simulink model "thinning1_131121"  (R2018b)
settings: Solver=FixedStepDiscrete  StartTime=0.0  StopTime=10.0  RelTol=1e-3
undefined symbols (not defined in the file or in its folder): gray
libraries: hdlsllib x2, visionsources x1, dspmtrx3 x1
settings Model: Creator=Administrator  LastModifiedBy=Administrator
settings OptimizationCC: BlockReduction=off  ConditionallyExecuteInputs=off  DefaultParameterBehavior=Inlined
settings DebuggingCC: AlgebraicLoopMsg=error  SingleTaskRateTransMsg=error
settings HardwareCC: ProdBitPerPointer=32  ProdBitPerSizeT=32  ProdBitPerPtrDiffT=32  ProdLargestAtomicFloat=None  ProdIntDivRoundTo=Undefined  ProdEndianess=Unspecified  ProdWordSize=32  ProdHWDeviceType=ASIC/FPGA->ASIC/FPGA  TargetBitPerPointer=64  TargetBitPerSizeT=64  TargetBitPerPtrDiffT=64  TargetLongLongMode=on  TargetIntDivRoundTo=Zero  TargetEndianess=LittleEndian  TargetWordSize=64  TargetHWDeviceType=Custom Processor->MATLAB Host Computer  ProdEqTarget=off

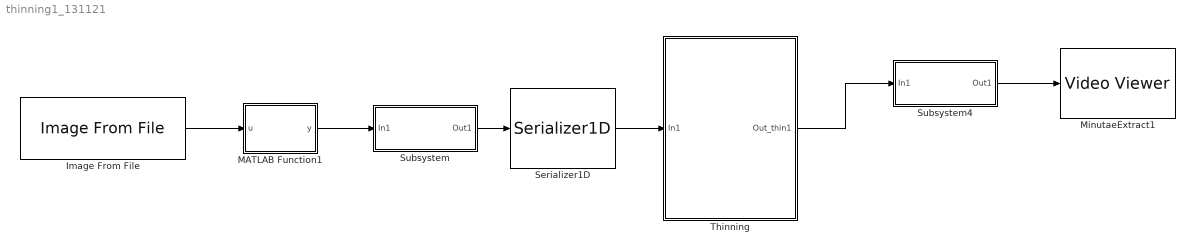
== system thinning1_131121 ==
  Image From File : visionsources/Image From File  Tag=vipblks_nd  FileName=C:\Users\Administrator\Desktop\chapter\101_4.tif  imagePorts=One multidimensional signal  Ts=0.1  ImageDataType=uint8  Signed=on  WordLength=16  sdImageDataType=uint(8)  FractionLengthMode=User-defined  FractionLength=15  OutPortLabels=R|G|B
      settings: SourceProductName=Computer Vision System Toolbox
  MATLAB Function1 : MATLAB Function  TreatAsAtomicUnit=on
  MinutaeExtract1 : VideoViewer  colormapValue=gray(256)  FigPos=[399 902 376 593]
  Serializer1D : hdlsllib/HDL Operations/Serializer1D  Ratio=1  IdleCycles=0  validIn=off  startOut=off  validOut=off  inputDataDimensions=8192  inputSampleTime=-1  inputSignalType=auto
      settings: SourceProductName=HDL Coder  SourceProductBaseCode=HD
  Subsystem : Subsystem
  Subsystem4 : Subsystem
  Thinning : Subsystem  TreatAsAtomicUnit=on
  wires:
  MATLAB Function1/1(y) -> Subsystem/1(In1)
  Image From File/1 -> MATLAB Function1/1(u)
  Subsystem/1(Out1) -> Serializer1D/1
  Serializer1D/1 -> Thinning/1(In1)
  Thinning/1(Out_thin1) -> Subsystem4/1(In1)
  Subsystem4/1(Out1) -> MinutaeExtract1/1

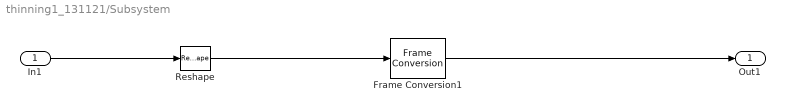
== system thinning1_131121/Subsystem ==
  In1 : Inport
  Frame Conversion1 : FrameConversion  OutFrame=Sample-based
  Reshape : Reshape
  Out1 : Outport
  wires:
  Frame Conversion1/1 -> Out1/1
  Reshape/1 -> Frame Conversion1/1
  In1/1 -> Reshape/1

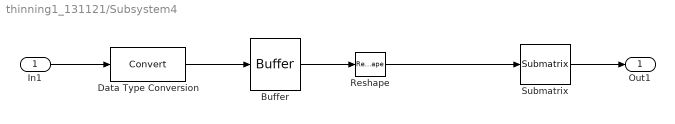
== system thinning1_131121/Subsystem4 ==
  In1 : Inport
  Buffer : Buffer  N=8192  OutputFrames=off
  Data Type Conversion : DataTypeConversion
  Reshape : Reshape  OutputDimensionality=Customize  OutputDimensions=[128,64]
  Submatrix : dspmtrx3/Submatrix  RowSpan=Range of rows  RowStartMode=First  RowStartIndex=1  RowEndMode=Last  RowEndIndex=1  ColSpan=Range of columns  ColStartMode=First  ColStartIndex=1  ColEndMode=Last  ColEndIndex=1
  Out1 : Outport
  wires:
  Data Type Conversion/1 -> Buffer/1
  Buffer/1 -> Reshape/1
  Reshape/1 -> Submatrix/1
  Submatrix/1 -> Out1/1
  In1/1 -> Data Type Conversion/1

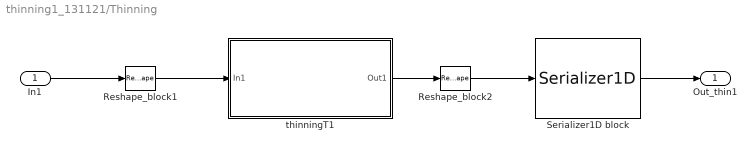
== system thinning1_131121/Thinning ==
  In1 : Inport
  Reshape_block1 : Reshape  OutputDimensionality=Customize  OutputDimensions=[128,64]
  Reshape_block2 : Reshape  OutputDimensionality=Column vector (2-D)  OutputDimensions=[128,64]
  Serializer1D block : hdlsllib/HDL Operations/Serializer1D  Ratio=8192  IdleCycles=0  validIn=off  startOut=off  validOut=off  inputDataDimensions=-1  inputSampleTime=-1  inputSignalType=auto
      settings: SourceProductName=HDL Coder  SourceProductBaseCode=HD
  thinningT1 : Subsystem  TreatAsAtomicUnit=on
  Out_thin1 : Outport
  wires:
  Reshape_block1/1 -> thinningT1/1(In1)
  In1/1 -> Reshape_block1/1
  Reshape_block2/1 -> Serializer1D block/1
  Serializer1D block/1 -> Out_thin1/1
  thinningT1/1(Out1) -> Reshape_block2/1

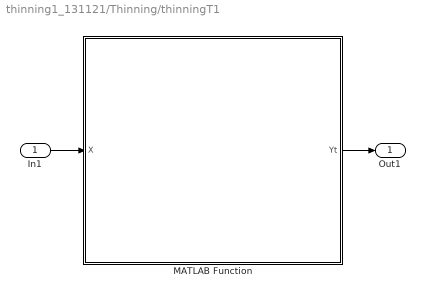
== system thinning1_131121/Thinning/thinningT1 ==
  In1 : Inport
  MATLAB Function : MATLAB Function  TreatAsAtomicUnit=on
  Out1 : Outport
  wires:
  In1/1 -> MATLAB Function/1(X)
  MATLAB Function/1(Yt) -> Out1/1

== matlab function thinning1_131121/MATLAB Function1 ==
  data: u input; y output
function y = fcn(u)
%#codegen
%i = rgb2gray(u);
b = u(100:227,150:213);
y = imbinarize(b);
%y = y(100:227,150:213);
%y = imbinarize(r);

== matlab function thinning1_131121/Thinning/thinningT1/MATLAB Function ==
  data: X input; Yt output
function Yt=thinningTh(X)
%img = imread ('2_4.jpg'); 
%Xr = rgb2gray(img);
%%%X = imbinarize(Xr);
%X = X(1:128,1:64);
[M,N]=size(X);
Yt = false(M,N);
Y=false(M,N,20);
Z=false(M,N,20);
Y(:,:,1)=X;
Z(:,:,1)=X;
for k=2:20
    Y(:,:,k)=Y(:,:,k-1);
    for i=2:M-1
        for j=2:N-1
            y11=Y(i-1,j-1,k);
            y12=Y(i-1,j,k);
            y13=Y(i-1,j+1,k);
            y21=Y(i,j-1,k);
            y22=Y(i,j,k);
            y23=Y(i,j+1,k);
            y31=Y(i+1,j-1,k);
            y32=Y(i+1,j,k);
            y33=Y(i+1,j+1,k);
            if y22==0
                if y11==1&&y12==1&&y13==1&&y31==0&&y32==0&&y33==0
                    Y(i,j,k)=1;
                elseif y11==1&&y13==0&&y21==1&&y23==0&&y31==1&&y33==0
                    Y(i,j,k)=1;
                elseif y11==0&&y12==0&&y13==0&&y31==1&&y32==1&&y33==1
                    Y(i,j,k)=1;
                elseif y11==0&&y13==1&&y21==0&&y23==1&&y31==0&&y33==1
                    Y(i,j,k)=1;
                elseif y12==1&&y13==1&&y21==0&&y23==1&&y32==0
                    Y(i,j,k)=1;
                elseif y11==1&&y12==1&&y21==1&&y23==0&&y32==0
                    Y(i,j,k)=1;
                elseif y12==0&&y21==1&&y23==0&&y31==1&&y21==1
                    Y(i,j,k)=1;
                elseif y12==0&&y21==0&&y23==1&&y32==1&&y33==1
                    Y(i,j,k)=1;
                    %extra
                elseif y11==0&&y12==0&&y23==1&&y31==1&&y32==1&&y33==1
                    Y(i,j,k)=1;
                end
            else
            end
        end
    end
%    Y(:,:,k)= Y(:,:,k-1);
     if Y(:,:,k)==Y(:,:,k-1)
%         break;
     end
end
Yt=Y(:,:,k);
%figure;
%imshow(Y);
